simulink subsystem "Distance_from_Speaker"  (R2023b)
settings: Solver=VariableStepAuto  StartTime=0.0  StopTime=10.0  RelTol=1e-3
undefined symbols (not defined in the file): AT_Tag_4_Coordinate_X, AT_Tag_4_Coordinate_Y, AT_Tag_7_Coordinate_X, AT_Tag_7_Coordinate_Y, TEST_Speaker_Distance
settings Model: Creator=ander  LastModifiedBy=ander

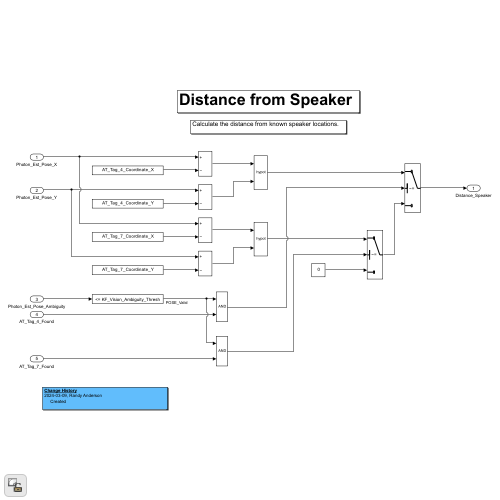
[thumbnail: Simulink's stored preview of the top-level diagram]
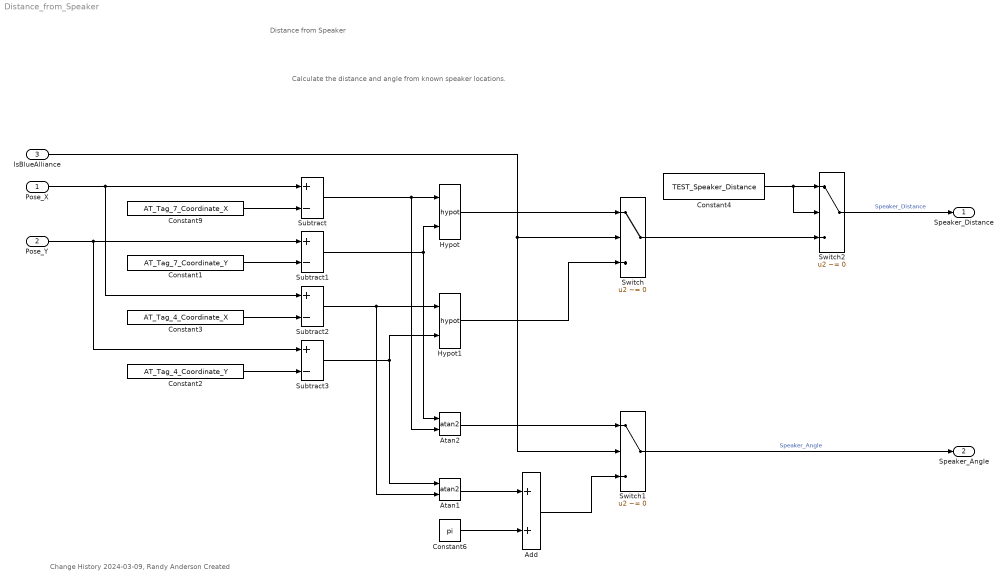
== system Distance_from_Speaker ==
  note: Distance from Speaker
  note: Calculate the distance and angle from known speaker locations.
  note: Change History
      | 2024-03-09, Randy Anderson
      | Created
  Pose_X : Inport
  Pose_Y : Inport  Port=2
  IsBlueAlliance : Inport  Port=3
  Add : Sum
  Atan1 : Trigonometry  Operator=atan2
  Atan2 : Trigonometry  Operator=atan2
  Constant1 : Constant  Value=AT_Tag_7_Coordinate_Y
  Constant2 : Constant  Value=AT_Tag_4_Coordinate_Y
  Constant3 : Constant  Value=AT_Tag_4_Coordinate_X
  Constant4 : Constant  Value=TEST_Speaker_Distance
  Constant6 : Constant  Value=pi
  Constant9 : Constant  Value=AT_Tag_7_Coordinate_X
  Hypot : Math  Operator=hypot
  Hypot1 : Math  Operator=hypot
  Subtract{,1..3} (4 alike) : Sum  Inputs=+-
  Switch : Switch  Criteria=u2 ~= 0  SaturateOnIntegerOverflow=off  InputSameDT=off
  Switch1 : Switch  Criteria=u2 ~= 0  SaturateOnIntegerOverflow=off  InputSameDT=off
  Switch2 : Switch  Criteria=u2 ~= 0  SaturateOnIntegerOverflow=off  InputSameDT=off
  Speaker_Distance : Outport
  Speaker_Angle : Outport  Port=2
  wires:
  Pose_X/1 -> Subtract2/1, Subtract/1
  Constant9/1 -> Subtract/2
  Pose_Y/1 -> Subtract3/1, Subtract1/1
  Constant1/1 -> Subtract1/2
  Constant3/1 -> Subtract2/2
  Constant2/1 -> Subtract3/2
  Subtract/1 -> Hypot/1, Atan2/2
  Subtract1/1 -> Atan2/1, Hypot/2
  Subtract2/1 -> Hypot1/1, Atan1/2
  Subtract3/1 -> Hypot1/2, Atan1/1
  Hypot/1 -> Switch/1
  Switch2/1 -> Speaker_Distance/1  "Speaker_Distance"
  Switch/1 -> Switch2/3
  Constant4/1 -> Switch2/1, Switch2/2
  IsBlueAlliance/1 -> Switch/2, Switch1/2
  Hypot1/1 -> Switch/3
  Atan2/1 -> Switch1/1
  Switch1/1 -> Speaker_Angle/1  "Speaker_Angle"
  Add/1 -> Switch1/3
  Atan1/1 -> Add/1
  Constant6/1 -> Add/2
